simulink model "cs_proj_ol_ramp"  (R2021b)
settings: Solver=ode4  StartTime=0.0  StopTime=10.0  FixedStep=0.001  RelTol=1e-3
libraries: simulink x1
settings Model: Creator=shash  LastModifiedBy=shash
settings DataIOCC: ReturnWorkspaceOutputs=off

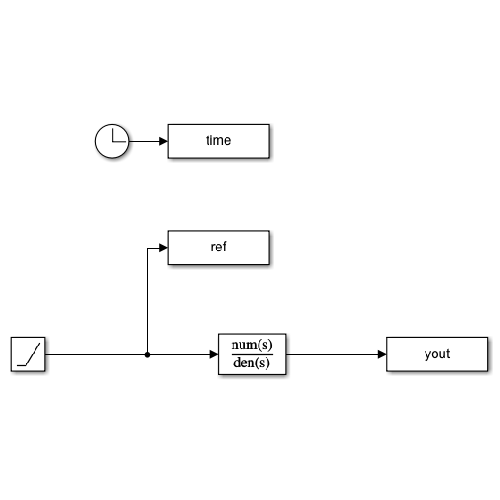
[thumbnail: Simulink's stored preview of the top-level diagram]
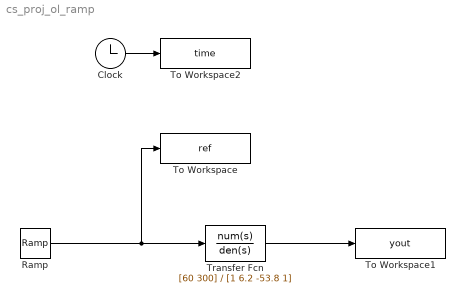
== system cs_proj_ol_ramp ==
  Clock : Clock
  Ramp : simulink/Sources/Ramp  slope=1  start=0  InitialOutput=0
  To Workspace : ToWorkspace  VariableName=ref  SampleTime=-1
  To Workspace1 : ToWorkspace  VariableName=yout  SampleTime=-1
  To Workspace2 : ToWorkspace  VariableName=time  SampleTime=-1
  Transfer Fcn : TransferFcn  Numerator=[60 300]  Denominator=[1 6.2 -53.8 1]
  wires:
  Ramp/1 -> To Workspace/1, Transfer Fcn/1
  Transfer Fcn/1 -> To Workspace1/1
  Clock/1 -> To Workspace2/1
